simulink model "FruitSorting_slice"  (R2025a)
settings: Solver=FixedStepDiscrete  StartTime=0.0  StopTime=0.01  FixedStep=0.002  RelTol=1e-3
settings Model: Creator=Mugin  LastModifiedBy=Mugin

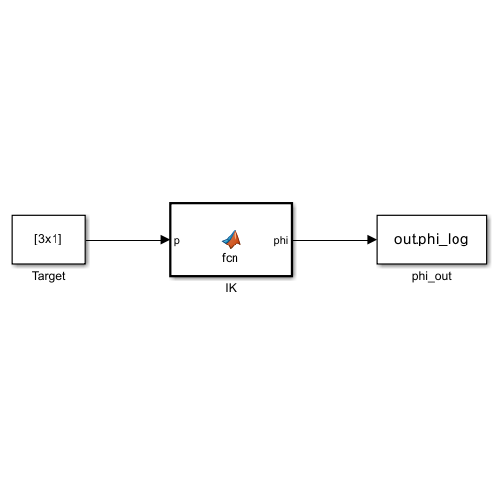
[thumbnail: Simulink's stored preview of the top-level diagram]
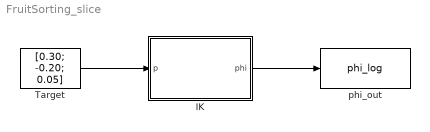
== system FruitSorting_slice ==
  IK : MATLAB Function  TreatAsAtomicUnit=on
  Target : Constant  Value=[0.30; -0.20; 0.05]  SampleTime=0.002
  phi_out : ToWorkspace  VariableName=phi_log  SampleTime=-1
  wires:
  Target/1 -> IK/1(p)
  IK/1(phi) -> phi_out/1

== matlab function FruitSorting_slice/IK ==
  data: p input; phi output
function phi = fcn(p)
%#codegen
coder.extrinsic('py_ik');
phi = zeros(4,1);
phi = py_ik(p);
end
